simulink model "dynamical_model_extended"  (R2017b)
settings: Solver=ode4  StartTime=0.0  StopTime=3  FixedStep=dt  RelTol=1e-3
undefined symbols (not defined in the file or in its folder): alpha0, c1, c2, c3, d0, dq_0, g, m, p_true, q_0, r
libraries: dspinverses x2
(part 1 of 3)
settings Model: Creator=s156443  LastModifiedBy=s156443

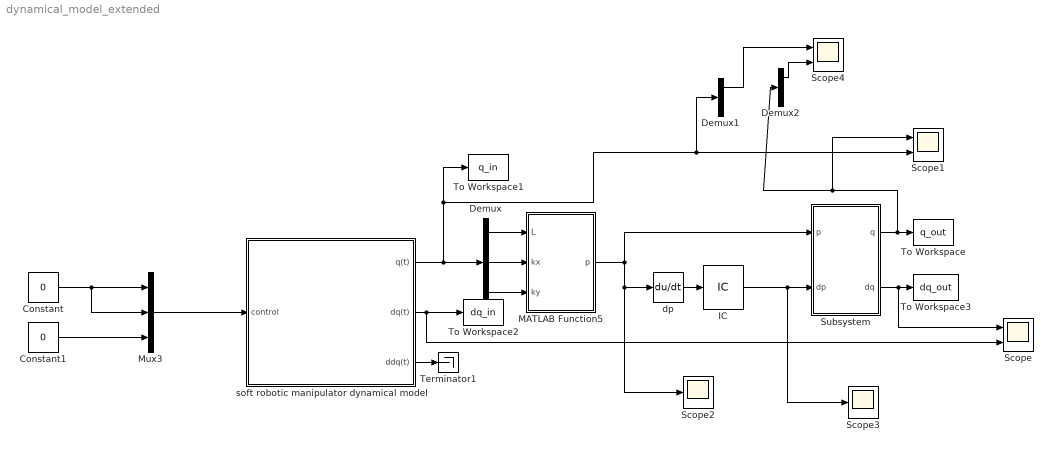
== system dynamical_model_extended ==
  Constant : Constant  Value=0
  Constant1 : Constant  Value=0
  Demux : Demux  Outputs=3
  Demux1 : Demux  Outputs=3
  Demux2 : Demux  Outputs=3
  IC : InitialCondition  Value=[1.3693551715, 0,0]
  MATLAB Function5 : MATLAB Function  TreatAsAtomicUnit=on
  Mux3 : Mux  Inputs=3
  Scope : Scope  NumInputPorts=2
  Scope1 : Scope  NumInputPorts=2
  Scope2 : Scope
  Scope3 : Scope
  Scope4 : Scope  NumInputPorts=2
  Subsystem : Subsystem
  Terminator1 : Terminator
  To Workspace : ToWorkspace  VariableName=q_out  SampleTime=-1
  To Workspace1 : ToWorkspace  VariableName=q_in  SampleTime=-1
  To Workspace2 : ToWorkspace  VariableName=dq_in  SampleTime=-1
  To Workspace3 : ToWorkspace  VariableName=dq_out  SampleTime=-1
  dp : Derivative
  soft robotic manipulator dynamical model : Subsystem
  wires:
  Constant/1 -> Mux3/2, Mux3/1
  Mux3/1 -> soft robotic manipulator dynamical model/1("control ")
  Constant1/1 -> Mux3/3
  Demux/1 -> MATLAB Function5/1(L)
  Demux/2 -> MATLAB Function5/2(kx)
  Demux/3 -> MATLAB Function5/3(ky)
  soft robotic manipulator dynamical model/1(q(t)) -> Demux/1, Demux1/1, Scope1/2, To Workspace1/1
  soft robotic manipulator dynamical model/3("ddq(t) ") -> Terminator1/1
  MATLAB Function5/1(p) -> Scope2/1, dp/1, Subsystem/1(p)
  Subsystem/1(q) -> Demux2/1, Scope1/1, To Workspace/1
  dp/1 -> IC/1
  soft robotic manipulator dynamical model/2("dq(t) ") -> To Workspace2/1, Scope/2
  Subsystem/2(dq) -> Scope/1, To Workspace3/1
  IC/1 -> Scope3/1, Subsystem/2(dp)
  Demux2/1 -> Scope4/2
  Demux1/1 -> Scope4/1

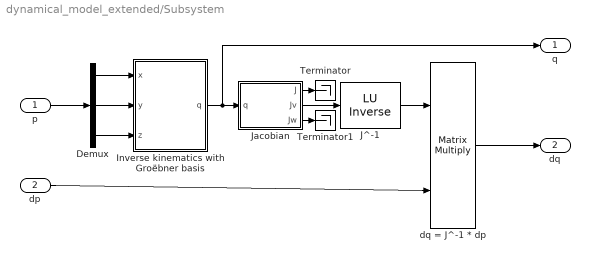
== system dynamical_model_extended/Subsystem ==
  p : Inport
  dp : Inport  Port=2
  " J^-1" : dspinverses/ LU Inverse
      settings: SourceProductName=DSP System Toolbox
  Demux : Demux  Outputs=3
  Inverse kinematics with Groëbner basis : MATLAB Function  TreatAsAtomicUnit=on
  "Jacobian " : MATLAB Function  TreatAsAtomicUnit=on
  Terminator : Terminator
  Terminator1 : Terminator
  dq = J^-1 * dp : Product  Multiplication=Matrix(*)
  q : Outport
  dq : Outport  Port=2
  wires:
  Inverse kinematics with Groëbner basis/1(q) -> q/1, "Jacobian "/1(q)
  "Jacobian "/2(Jv) -> " J^-1"/1
  " J^-1"/1 -> dq = J^-1 * dp/1
  dp/1 -> dq = J^-1 * dp/2
  dq = J^-1 * dp/1 -> dq/1
  "Jacobian "/1(J) -> Terminator/1
  "Jacobian "/3(Jw) -> Terminator1/1
  Demux/2 -> Inverse kinematics with Groëbner basis/2(y)
  Demux/1 -> Inverse kinematics with Groëbner basis/1(x)
  Demux/3 -> Inverse kinematics with Groëbner basis/3(z)
  p/1 -> Demux/1

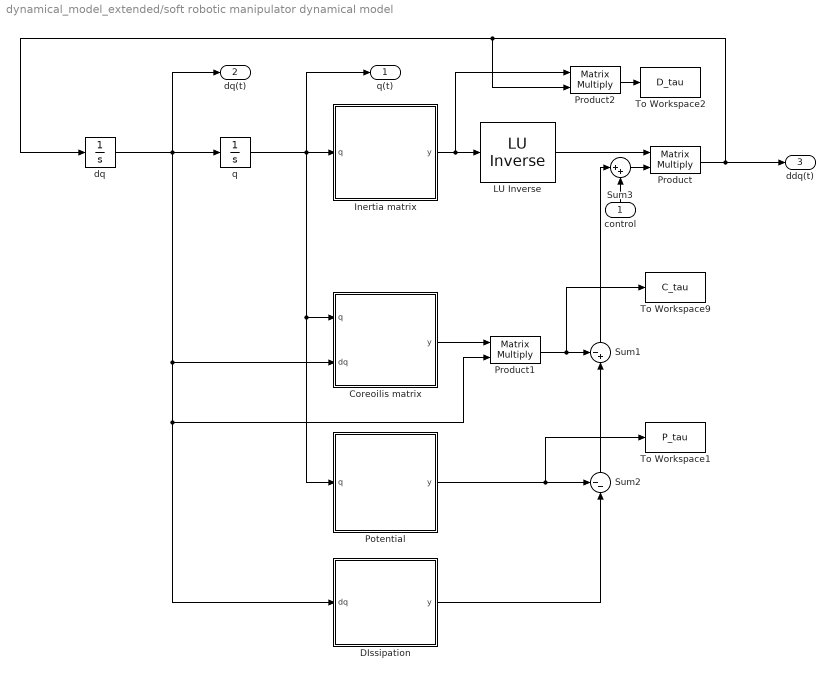
== system dynamical_model_extended/soft robotic manipulator dynamical model ==
  "control " : Inport
  " LU Inverse" : dspinverses/ LU Inverse
      settings: SourceProductName=DSP System Toolbox
  "Coreoilis matrix " : MATLAB Function  TreatAsAtomicUnit=on
  "DIssipation " : MATLAB Function  TreatAsAtomicUnit=on
  "Inertia matrix " : MATLAB Function  TreatAsAtomicUnit=on
  Potential : MATLAB Function  TreatAsAtomicUnit=on
  Product : Product  Multiplication=Matrix(*)
  Product1 : Product  Multiplication=Matrix(*)
  Product2 : Product  Multiplication=Matrix(*)
  Sum1 : Sum  Inputs=-+|
  Sum2 : Sum  Inputs=--|
  Sum3 : Sum  Inputs=|++
  To Workspace1 : ToWorkspace  VariableName=P_tau  SampleTime=-1
      settings: Save2DSignal=2-D array (concatenate along first dimension)
  To Workspace2 : ToWorkspace  VariableName=D_tau  SampleTime=-1
      settings: Save2DSignal=2-D array (concatenate along first dimension)
  To Workspace9 : ToWorkspace  VariableName=C_tau  SampleTime=-1
      settings: Save2DSignal=2-D array (concatenate along first dimension)
  dq : Integrator  InitialCondition=dq_0
  q : Integrator  InitialCondition=q_0
  q(t) : Outport
  "dq(t) " : Outport  Port=2
  "ddq(t) " : Outport  Port=3
  wires:
  "Inertia matrix "/1(y) -> Product2/1, " LU Inverse"/1
  " LU Inverse"/1 -> Product/1
  Potential/1(y) -> To Workspace1/1, Sum2/1
  Sum2/1 -> Sum1/2
  dq/1 -> "dq(t) "/1, q/1, "Coreoilis matrix "/2(dq), "DIssipation "/1(dq), Product1/2
  "control "/1 -> Sum3/2
  "DIssipation "/1(y) -> Sum2/2
  "Coreoilis matrix "/1(y) -> Product1/1
  Sum3/1 -> Product/2
  Product/1 -> "ddq(t) "/1, Product2/2, dq/1
  Sum1/1 -> Sum3/1
  q/1 -> "Inertia matrix "/1(q), q(t)/1, "Coreoilis matrix "/1(q), Potential/1(q)
  Product2/1 -> To Workspace2/1
  Product1/1 -> Sum1/1, To Workspace9/1
